simulink model "dummy"  (R2018b)
settings: Solver=VariableStepAuto  StartTime=0.0  StopTime=0  RelTol=1e-3
values from neighbouring files (symbols this model uses):
  nodePos = [R1_o init_Ri_o Rn_o]    [tester2.m]
  nodeVel = zeros(size(nodePos))    [tester2.m]
  sumF = fGrav + nodeDrag + nodeTen    [calcTetForce.m]
  tetLength = 95    [tester2.m]
  Vflow = [1;0]    [tester2.m]
libraries: planarTether_ul x1
settings Model: Creator=Ayaz  LastModifiedBy=Ayaz

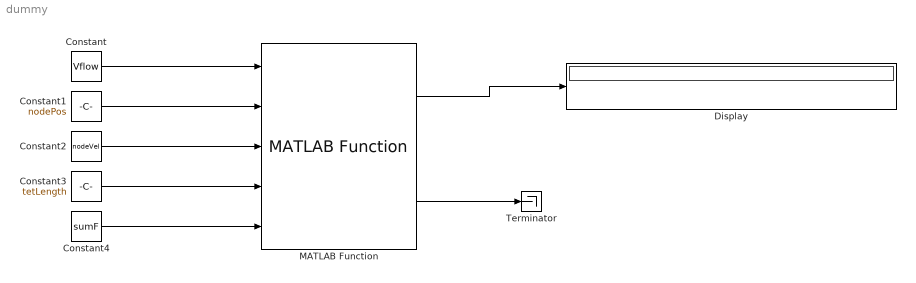
== system dummy ==
  Constant : Constant  Value=Vflow  VectorParams1D=off
  Constant1 : Constant  Value=nodePos  VectorParams1D=off
  Constant2 : Constant  Value=nodeVel  VectorParams1D=off
  Constant3 : Constant  Value=tetLength  VectorParams1D=off
  Constant4 : Constant  Value=sumF  VectorParams1D=off
  Display : Display
  MATLAB Function : planarTether_ul/planarTether/MATLAB Function  SystemSampleTime=-1
  Terminator : Terminator
  wires:
  Constant1/1 -> MATLAB Function/2
  Constant2/1 -> MATLAB Function/3
  Constant3/1 -> MATLAB Function/4
  Constant4/1 -> MATLAB Function/5
  Constant/1 -> MATLAB Function/1
  MATLAB Function/1 -> Display/1
  MATLAB Function/2 -> Terminator/1
